simulink library "Lib_Piccolo"  (R2018b)
settings: Solver=VariableStepAuto  StartTime=0.0  StopTime=10.0  RelTol=1e-3
values from neighbouring files (symbols this model uses):
  AccelErrInt2Brakes = 0.15    [SimulationControlConfig16P.m]    (also in SimulationControlConfig16P_F0.m; SimulationControlConfig16P_F2.m; SimulationControlConfig16P_LEGACY.m; SimulationControlConfigTAILLESS.m = 0.2)
  AileronMax = 25    [SimulationControlConfig16P.m]    (also in SimulationControlConfig16P_F0.m; SimulationControlConfig16P_F2.m; SimulationControlConfig16P_LEGACY.m; SimulationControlConfigTAILLESS.m)
  AileronPower = 0.00268    [SimulationControlConfig16P.m]    (also in SimulationControlConfig16P_F0.m; SimulationControlConfig16P_F2.m; SimulationControlConfig16P_LEGACY.m; SimulationControlConfigTAILLESS.m = 0.002266)
  AileronSurfaceMax = 45    [SimulationControlConfig16P.m]    (also in SimulationControlConfig16P_F0.m; SimulationControlConfig16P_F2.m; SimulationControlConfig16P_LEGACY.m; SimulationControlConfigTAILLESS_CGAFT_F0.m = 25)
  AileronTrim = 0    [SimulationControlConfig16P.m]    (also in SimulationControlConfig16P_F0.m; SimulationControlConfig16P_F2.m; SimulationControlConfig16P_LEGACY.m; SimulationControlConfigTAILLESS.m)
  Alt = 1000 + TerrainHeight    [SimulationStateConfig.m]
  AltCruise_m = Alt * 0.3048    [SimulationControlConfig16P.m]    (also in SimulationControlConfig16P_F2.m; SimulationControlConfigTAILLESS.m = Alt/3.28084; SimulationControlConfigTAILLESS_CGAFT_F0.m = 640; SimulationControlConfigTAILLESS_CGFWD_F0.m = 640)
  AltitudeRate2PitchCmdIntegratorInit = 0.1    [SimulationControlPre.m]
  AltMax = 10000    [SimulationControlConfig16P.m]    (also in SimulationControlConfig16P_F0.m; SimulationControlConfig16P_F2.m; SimulationControlConfig16P_LEGACY.m; SimulationControlConfigTAILLESS.m)
  AltMaxAccel = 2.5    [SimulationControlConfig16P.m]    (also in SimulationControlConfig16P_F0.m = 2; SimulationControlConfig16P_F2.m = 2; SimulationControlConfig16P_LEGACY.m = 0.9; SimulationControlConfigTAILLESS.m = 2)
  AltMin = 0    [SimulationControlConfig16P.m]    (also in SimulationControlConfig16P_F0.m; SimulationControlConfig16P_F2.m; SimulationControlConfig16P_LEGACY.m; SimulationControlConfigTAILLESS.m)
  AltRateCmd2Pitch = 0.26    [SimulationControlConfig16P.m]    (also in SimulationControlConfig16P_F0.m = 0.35; SimulationControlConfig16P_F2.m = 0.35; SimulationControlConfig16P_LEGACY.m = 0.6; SimulationControlConfigTAILLESS.m = 0.9)
  AltRateError2Pitch = 0.34    [SimulationControlConfig16P.m]    (also in SimulationControlConfig16P_F0.m = 0.61; SimulationControlConfig16P_F2.m = 0.61; SimulationControlConfig16P_LEGACY.m = 0.4; SimulationControlConfigTAILLESS.m = 0.3)
  AltRateErrorInt2Pitch = 0.61    [SimulationControlConfig16P.m]    (also in SimulationControlConfig16P_F0.m = 0.28; SimulationControlConfig16P_F2.m = 0.28; SimulationControlConfig16P_LEGACY.m = 0.45; SimulationControlConfigTAILLESS.m = 0.15)
  AltRateLpfCutOff = 3    [SimulationControlConfig16P.m]    (also in SimulationControlConfig16P_F0.m; SimulationControlConfig16P_F2.m; SimulationControlConfig16P_LEGACY.m; SimulationControlConfigTAILLESS.m = 5)
  AutoNosegear2Rudder = 26    [SimulationControlConfig16P.m]    (also in SimulationControlConfig16P_F0.m; SimulationControlConfig16P_F2.m; SimulationControlConfig16P_LEGACY.m; SimulationControlConfigTAILLESS.m = 25.2)
  b = 5.54    [SimulationControlConfig16P.m]    (also in SimulationControlConfig16P_F0.m; SimulationControlConfig16P_F2.m; SimulationControlConfig16P_LEGACY.m; SimulationControlConfigTAILLESS.m = 2.37)
  Bank2AileronIntegratorInit = 0    [SimulationControlPre.m]
  BankMax_User = BankMax_User/180*pi    (= 0.610865238198)    [SimulationControlConfig16P.m]    (also in SimulationControlConfig16P_F0.m = 0.523598775598; SimulationControlConfig16P_F2.m = 0.523598775598; SimulationControlConfig16P_LEGACY.m = 0.523598775598; SimulationControlConfigTAILLESS.m = 0.558505360638)
  baseLegFlaps = 20    [SimulationControlConfig16P.m]    (also in SimulationControlConfig16P_F0.m; SimulationControlConfig16P_F2.m = 15; SimulationControlConfig16P_LEGACY.m = 0; SimulationControlConfigTAILLESS.m = 0)
  C = GeneticOpt.C    [SimulationCostFunction.m]
  c = Sw/b    (= 0.841696750903)    [SimulationControlConfig16P.m]    (also in SimulationControlConfig16P_F0.m; SimulationControlConfig16P_F2.m; SimulationControlConfig16P_LEGACY.m; SimulationControlConfigTAILLESS.m = 0.354008438819)
  cell2WheelFactorMG = 5.98    [SimulationSensorConfig16P_LEGACY.m]
  cell2WheelFactorNG = 1    [SimulationSensorConfig16P_LEGACY.m]
  cellSatMaxMG = 15000    [SimulationSensorConfig16P.m]    (also in SimulationSensorConfig16P_LEGACY.m; SimulationSensorConfigTAILLESS7P.m; SimulationSensorConfigUTAIL7P.m)
  cellSatMaxNG = 1000    [SimulationSensorConfig16P.m]    (also in SimulationSensorConfig16P_LEGACY.m; SimulationSensorConfigTAILLESS7P.m; SimulationSensorConfigUTAIL7P.m)
  cellSatMinMG = -15000    [SimulationSensorConfig16P.m]    (also in SimulationSensorConfig16P_LEGACY.m; SimulationSensorConfigTAILLESS7P.m; SimulationSensorConfigUTAIL7P.m)
  cellSatMinNG = -1000    [SimulationSensorConfig16P.m]    (also in SimulationSensorConfig16P_LEGACY.m; SimulationSensorConfigTAILLESS7P.m; SimulationSensorConfigUTAIL7P.m)
  CL_Limit = CL_Max    (= 0.54)    [SimulationControlConfig16P.m]    (also in SimulationControlConfig16P_F0.m; SimulationControlConfig16P_F2.m = 0.638; SimulationControlConfig16P_LEGACY.m; SimulationControlConfigTAILLESS.m = 0.525)
  CL_Max = 0.54    [SimulationControlConfig16P.m]    (also in SimulationControlConfig16P_F0.m; SimulationControlConfig16P_F2.m = 0.638; SimulationControlConfig16P_LEGACY.m; SimulationControlConfigTAILLESS.m = 0.525)
  CL_Max_Nom = 0.465    [SimulationControlConfig16P.m]    (also in SimulationControlConfig16P_F0.m; SimulationControlConfig16P_F2.m = 0.563; SimulationControlConfig16P_LEGACY.m; SimulationControlConfigTAILLESS.m = 0.39)
  CL_Min = 0    [SimulationControlConfig16P.m]    (also in SimulationControlConfig16P_F0.m; SimulationControlConfig16P_F2.m; SimulationControlConfig16P_LEGACY.m; SimulationControlConfigTAILLESS.m)
  ClimbMaxFraction = 0.35    [SimulationControlConfig16P.m]    (also in SimulationControlConfig16P_F0.m = 0.17; SimulationControlConfig16P_F2.m = 0.17; SimulationControlConfig16P_LEGACY.m = 0.24; SimulationControlConfigTAILLESS.m = 0.21)
  ClimboutMaxBank = 7.0    (= 7)    [SimulationControlConfig16P.m]    (also in SimulationControlConfig16P_F0.m; SimulationControlConfig16P_F2.m; SimulationControlConfig16P_LEGACY.m; SimulationControlConfigTAILLESS.m = 5)
  ClimboutTimer = 7.0    (= 7)    [SimulationControlConfig16P.m]    (also in SimulationControlConfig16P_F0.m; SimulationControlConfig16P_F2.m; SimulationControlConfig16P_LEGACY.m; SimulationControlConfigTAILLESS.m)
  dCl_per_dFlap = 0.005581818    [SimulationControlConfig16P.m]    (also in SimulationControlConfig16P_F0.m = 0; SimulationControlConfig16P_F2.m = 0.0065; SimulationControlConfig16P_LEGACY.m = 0; SimulationControlConfigTAILLESS.m = 0)
  DecelerationCmd = 3.1    [SimulationControlConfig16P.m]    (also in SimulationControlConfig16P_F0.m; SimulationControlConfig16P_F2.m; SimulationControlConfig16P_LEGACY.m; SimulationControlConfigTAILLESS.m = 0.1)
  DeRotateLogicEndTimer = abs((NoseDownLimit_Deg-1)/DeRotateRamp_Dps)    [SimulationControlConfig16P.m]    (also in SimulationControlConfig16P_F0.m; SimulationControlConfig16P_F2.m; SimulationControlConfig16P_LEGACY.m; SimulationControlConfigTAILLESS.m)
  DeRotateLogicHoldNoseUpTimer = 0.1    [SimulationControlConfig16P.m]    (also in SimulationControlConfig16P_F0.m; SimulationControlConfig16P_F2.m; SimulationControlConfig16P_LEGACY.m; SimulationControlConfigTAILLESS.m)
  DeRotateLogicTimerTimeout = 2    [SimulationControlConfig16P.m]    (also in SimulationControlConfig16P_F0.m; SimulationControlConfig16P_F2.m; SimulationControlConfig16P_LEGACY.m; SimulationControlConfigTAILLESS.m)
  DeRotateLowerCmdSaturation = 0    [SimulationControlConfig16P.m]    (also in SimulationControlConfig16P_F0.m; SimulationControlConfig16P_F2.m; SimulationControlConfig16P_LEGACY.m; SimulationControlConfigTAILLESS.m)
  DeRotateRamp_Dps = 3    [SimulationControlConfig16P.m]    (also in SimulationControlConfig16P_F0.m; SimulationControlConfig16P_F2.m; SimulationControlConfig16P_LEGACY.m; SimulationControlConfigTAILLESS.m = 8)
  DeRotateUpperCmdSaturation = 7    [SimulationControlConfig16P.m]    (also in SimulationControlConfig16P_F0.m; SimulationControlConfig16P_F2.m; SimulationControlConfig16P_LEGACY.m; SimulationControlConfigTAILLESS.m)
  DescentMaxFraction = 0.22    [SimulationControlConfig16P.m]    (also in SimulationControlConfig16P_F0.m = 0.2; SimulationControlConfig16P_F2.m = 0.2; SimulationControlConfig16P_LEGACY.m = 0.2; SimulationControlConfigTAILLESS.m = 0.17)
  DesktopSimTerrainOffset_m = 0.406    [SimulationAircraftConfig.m]
  downwindFlaps = 0    [SimulationControlConfig16P.m]    (also in SimulationControlConfig16P_F0.m; SimulationControlConfig16P_F2.m = 15; SimulationControlConfig16P_LEGACY.m; SimulationControlConfigTAILLESS.m)
  downwindSplitAil = 0    [SimulationControlConfig16P_F2.m]
  DP_init = 0.5*1.225*V_init^2    [SimulationControlConfig16P.m]    (also in SimulationControlConfig16P_F0.m; SimulationControlConfig16P_F2.m; SimulationControlConfig16P_LEGACY.m; SimulationControlConfigTAILLESS.m)
  dscNoiseMG = 1    [SimulationSensorConfig16P_LEGACY.m]
  dscNoiseNG = 0.25    [SimulationSensorConfig16P_LEGACY.m]
  DSCnumBits = 24    [SimulationSensorConfig16P.m]    (also in SimulationSensorConfig16P_LEGACY.m; SimulationSensorConfigTAILLESS7P.m; SimulationSensorConfigUTAIL7P.m)
  DSCRangeMaxMG = 15000    [SimulationSensorConfig16P.m]    (also in SimulationSensorConfig16P_LEGACY.m; SimulationSensorConfigTAILLESS7P.m; SimulationSensorConfigUTAIL7P.m)
  DSCRangeMaxNG = 1000    [SimulationSensorConfig16P.m]    (also in SimulationSensorConfig16P_LEGACY.m; SimulationSensorConfigTAILLESS7P.m; SimulationSensorConfigUTAIL7P.m)
  DSCRangeMinMG = -15000    [SimulationSensorConfig16P.m]    (also in SimulationSensorConfig16P_LEGACY.m; SimulationSensorConfigTAILLESS7P.m; SimulationSensorConfigUTAIL7P.m)
  DSCRangeMinNG = -1000    [SimulationSensorConfig16P.m]    (also in SimulationSensorConfig16P_LEGACY.m; SimulationSensorConfigTAILLESS7P.m; SimulationSensorConfigUTAIL7P.m)
  dt = DLLSim.dt    [SimulationTimeStep.m]    (also in SimulationTrim.m = 0.02)
  EarlyTouchdownThreshold = 3.0    (= 3)    [SimulationControlConfig16P.m]    (also in SimulationControlConfig16P_F0.m; SimulationControlConfig16P_F2.m; SimulationControlConfig16P_LEGACY.m; SimulationControlConfigTAILLESS.m)
  ElevatorDeflectionRate = 15    [SimulationControlConfig16P.m]    (also in SimulationControlConfig16P_F0.m; SimulationControlConfig16P_F2.m; SimulationControlConfig16P_LEGACY.m = 12; SimulationControlConfigTAILLESS.m = 5)
  ElevatorMax = 25    [SimulationControlConfig16P.m]    (also in SimulationControlConfig16P_F0.m; SimulationControlConfig16P_F2.m; SimulationControlConfig16P_LEGACY.m; SimulationControlConfigTAILLESS.m)
  ElevatorPower = -0.002209    [SimulationControlConfig16P.m]    (also in SimulationControlConfig16P_F0.m; SimulationControlConfig16P_F2.m; SimulationControlConfig16P_LEGACY.m; SimulationControlConfigTAILLESS.m = -0.002668)
  ElevatorTrim = -3.5    [SimulationControlConfig16P.m]    (also in SimulationControlConfig16P_F0.m; SimulationControlConfig16P_F2.m; SimulationControlConfig16P_LEGACY.m; SimulationControlConfigTAILLESS.m = -3)
  elevonBias = 0    [SimulationControlConfig16P.m]    (also in SimulationControlConfig16P_F0.m; SimulationControlConfig16P_F2.m; SimulationControlConfig16P_LEGACY.m; SimulationControlConfigTAILLESS.m)
  Enable_TAS_Protection = 0    [SimulationControlConfig16P.m]    (also in SimulationControlConfig16P_F0.m; SimulationControlConfig16P_F2.m; SimulationControlConfig16P_LEGACY.m; SimulationControlConfigTAILLESS.m)
  EnableCrossTrackAbort = 1    [SimulationControlConfig16P.m]    (also in SimulationControlConfigTAILLESS.m; SimulationControlConfigTAILLESS_CGAFT_F0.m; SimulationControlConfigTAILLESS_CGFWD_F0.m; SimulationControlConfigTAILLESS_CGFWD_F2.m)
  EnergyBandwidth = 0.04    [SimulationControlConfig16P.m]    (also in SimulationControlConfig16P_F0.m = 0.03; SimulationControlConfig16P_F2.m = 0.03; SimulationControlConfig16P_LEGACY.m = 0.02; SimulationControlConfigTAILLESS.m = 0.06)
  EngineLhFuelCut = 0    [SimulationAircraftConfig.m]
  EngineRhFuelCut = 0    [SimulationAircraftConfig.m]
  FastThrottleRate = 0.075    [SimulationControlConfig16P.m]    (also in SimulationControlConfig16P_F0.m = 0.05; SimulationControlConfig16P_F2.m = 0.05; SimulationControlConfig16P_LEGACY.m = 0.05; SimulationControlConfigTAILLESS.m = 0.1)
  FilterWarmUpTime = 2    [SimulationSensorConfig16P.m]    (also in SimulationSensorConfig16P_LEGACY.m; SimulationSensorConfigTAILLESS7P.m; SimulationSensorConfigUTAIL7P.m)
  finalApproachFlaps = 20    [SimulationControlConfig16P.m]    (also in SimulationControlConfig16P_F0.m; SimulationControlConfig16P_F2.m = 15; SimulationControlConfig16P_LEGACY.m = 0; SimulationControlConfigTAILLESS.m = 0)
  finalApproachSplitAil = 20    [SimulationControlConfig16P_F2.m]
  FinalDescentSlope_Deg = testPlans(testIndx).descentSlope    [SimulationControlConfig16P.m]    (also in SimulationControlConfig16P_F0.m; SimulationControlConfig16P_F2.m; SimulationControlConfig16P_LEGACY.m; SimulationControlConfigTAILLESS.m)
  flapMax = 0    [SimulationControlConfig16P.m]    (also in SimulationControlConfig16P_F0.m = 35; SimulationControlConfig16P_F2.m = 33; SimulationControlConfig16P_LEGACY.m; SimulationControlConfigTAILLESS.m)
  flapRate = 7.5    [SimulationControlConfig16P.m]    (also in SimulationControlConfig16P_F0.m; SimulationControlConfig16P_F2.m; SimulationControlConfig16P_LEGACY.m; SimulationControlConfigTAILLESS.m = 6.6)
  FlareHeight = 5    [SimulationControlConfig16P.m]    (also in SimulationControlConfig16P_F0.m; SimulationControlConfig16P_F2.m; SimulationControlConfig16P_LEGACY.m = 4.8; SimulationControlConfigTAILLESS.m = 2.75)
  FlareVerticalRate_mps = -0.4    [SimulationControlConfig16P.m]    (also in SimulationControlConfig16P_F0.m; SimulationControlConfig16P_F2.m; SimulationControlConfig16P_LEGACY.m = -0.5; SimulationControlConfigTAILLESS.m = -0.15)
  Fp_Aileron = 0.55*2*pi*RollRateLpfCutoff*dt    [SimulationControlConfig16P.m]    (also in SimulationControlConfig16P_F0.m; SimulationControlConfig16P_F2.m; SimulationControlConfig16P_LEGACY.m; SimulationControlConfigTAILLESS.m)
  Fp_Alt = 2*pi*0.55*AltBandwidth    (= 0.622035345411)    [SimulationControlConfig16P.m]    (also in SimulationControlConfig16P_F0.m; SimulationControlConfig16P_F2.m; SimulationControlConfig16P_LEGACY.m = 0.099; SimulationControlConfigTAILLESS.m = 0.207345115137)
  Fp_AltRate = 0.55*2*pi*AltRateLpfCutOff*dt    [SimulationControlConfig16P.m]    (also in SimulationControlConfig16P_F0.m; SimulationControlConfig16P_F2.m; SimulationControlConfig16P_LEGACY.m; SimulationControlConfigTAILLESS.m)
  Fp_Elevator = 0.55*2*pi*PitchRateLpfCutoff*dt    [SimulationControlConfig16P.m]    (also in SimulationControlConfig16P_F0.m; SimulationControlConfig16P_F2.m; SimulationControlConfig16P_LEGACY.m; SimulationControlConfigTAILLESS.m)
  Fp_Energy = 0.55*2*pi*EnergyBandwidth    (= 0.138230076758)    [SimulationControlConfig16P.m]    (also in SimulationControlConfig16P_F0.m = 0.103672557568; SimulationControlConfig16P_F2.m = 0.103672557568; SimulationControlConfig16P_LEGACY.m = 0.069115038379; SimulationControlConfigTAILLESS.m = 0.207345115137)
  Fp_Energy2 = 0.55*2*pi*EnergyBandwidth*dt    [SimulationControlConfig16P.m]    (also in SimulationControlConfig16P_F0.m; SimulationControlConfig16P_F2.m; SimulationControlConfig16P_LEGACY.m; SimulationControlConfigTAILLESS.m)
  Fp_Pitch = 0.55*2*pi*PitchBandwidth    (= 2.45358386245)    [SimulationControlConfig16P.m]    (also in SimulationControlConfig16P_F0.m; SimulationControlConfig16P_F2.m = 1.72787595947; SimulationControlConfig16P_LEGACY.m = 3.11017672705; SimulationControlConfigTAILLESS.m = 1.55508836353)
  Fp_Pitch_2 = 0.55*2*pi*PitchBandwidth*dt    [SimulationControlConfig16P.m]    (also in SimulationControlConfig16P_F0.m; SimulationControlConfig16P_F2.m; SimulationControlConfig16P_LEGACY.m; SimulationControlConfigTAILLESS.m)
  Fp_Roll = RollBandwidth^2    (= 1.69)    [SimulationControlConfig16P.m]    (also in SimulationControlConfig16P_F0.m = 1.44; SimulationControlConfig16P_F2.m = 1.44; SimulationControlConfig16P_LEGACY.m = 1.44; SimulationControlConfigTAILLESS.m = 1.21)
  Fp_Rudder = 0.55*2*pi*YawRateLpfCutoff*dt    [SimulationControlConfig16P.m]    (also in SimulationControlConfig16P_F0.m; SimulationControlConfig16P_F2.m; SimulationControlConfig16P_LEGACY.m; SimulationControlConfigTAILLESS.m)
  Fp_TAS = 0.55*2*pi*TASBandwidth    (= 0.103672557568)    [SimulationControlConfig16P.m]    (also in SimulationControlConfig16P_F0.m; SimulationControlConfig16P_F2.m; SimulationControlConfig16P_LEGACY.m; SimulationControlConfigTAILLESS.m = 0.172787595947)
  Fp_TAS_Filter = 2*pi*TasLpfCutoff*dt    [SimulationControlConfig16P.m]    (also in SimulationControlConfig16P_F0.m; SimulationControlConfig16P_F2.m; SimulationControlConfig16P_LEGACY.m; SimulationControlConfigTAILLESS.m)
  Fp_Turn = 0.55*2*pi*TurnErrLPFcutoff    (= 0.172787595947)    [SimulationControlConfig16P.m]    (also in SimulationControlConfig16P_F0.m = 0.0345575191895; SimulationControlConfig16P_F2.m = 0.0345575191895; SimulationControlConfig16P_LEGACY.m = 0.0345575191895; SimulationControlConfigTAILLESS.m)
  Fp_TurnDerr = 0.55*2*pi*TurnDerivativeLPFcutoff    (= 0.172787595947)    [SimulationControlConfig16P.m]    (also in SimulationControlConfig16P_F0.m = 0.0345575191895; SimulationControlConfig16P_F2.m = 0.0345575191895; SimulationControlConfig16P_LEGACY.m = 0.0345575191895; SimulationControlConfigTAILLESS.m)
  FTV = 3    [SimulationAircraftConfig.m]
  ftvStaticPositionError = 1/1.18    (= 0.847457627119)    [SimulationSensorConfig16P.m]    (also in SimulationSensorConfig16P_LEGACY.m; SimulationSensorConfigTAILLESS7P.m = 1; SimulationSensorConfigUTAIL7P.m = 1)
  g = 9.81    [SimulationStateConfig.m]
  goAroundSplitAil = 0    [SimulationControlConfig16P_F2.m]
  GustSpd_Kts = testPlans(testIndx).gustSpd    [SimulationStateConfig.m]
  GustTriggerVal = testPlans(testIndx).gustTriggerVal    [SimulationStateConfig.m]
  HeadingErr2TurnRate = 0.5    [SimulationControlConfig16P.m]    (also in SimulationControlConfig16P_F0.m; SimulationControlConfig16P_F2.m; SimulationControlConfig16P_LEGACY.m; SimulationControlConfigTAILLESS.m)
  HeadingErrDer2TurnRate = 0.3    [SimulationControlConfig16P.m]    (also in SimulationControlConfig16P_F0.m; SimulationControlConfig16P_F2.m; SimulationControlConfig16P_LEGACY.m; SimulationControlConfigTAILLESS.m)
  IASbounce = IASstall*0.8    [SimulationControlPre.m]
  IAScruiseCMD = sqrt(2*m*9.81/(1.225*Sw*CL_cruise))    [SimulationControlConfig16P.m]    (also in SimulationControlConfig16P_F0.m; SimulationControlConfig16P_F2.m; SimulationControlConfig16P_LEGACY.m; SimulationControlConfigTAILLESS.m)
  IASfinalCMD = 1.12 * IASmin    [SimulationControlConfig16P.m]    (also in SimulationControlConfig16P_F0.m = 1.14 * IASmin; SimulationControlConfig16P_F2.m = 1.10 * IASmin; SimulationControlConfig16P_LEGACY.m = 1.10 * IASmin; SimulationControlConfigTAILLESS.m = 1.14 * IASmin)
  IASflareCMD = IASstall    [SimulationControlConfig16P.m]    (also in SimulationControlConfig16P_F0.m; SimulationControlConfig16P_F2.m; SimulationControlConfig16P_LEGACY.m; SimulationControlConfigTAILLESS.m)
  IASmax = 64    [SimulationControlConfig16P.m]    (also in SimulationControlConfig16P_F0.m = 46; SimulationControlConfig16P_F2.m = 52; SimulationControlConfig16P_LEGACY.m = 46; SimulationControlConfigTAILLESS.m = 38.9)
  IASmin = sqrt(2*m*9.81/(1.225*Sw*0.9*CL_Max_Nom))    [SimulationControlConfig16P.m]    (also in SimulationControlConfig16P_F0.m; SimulationControlConfig16P_F2.m; SimulationControlConfig16P_LEGACY.m; SimulationControlConfigTAILLESS.m)
  IASshortCMD = IASstall    [SimulationControlConfig16P.m]    (also in SimulationControlConfig16P_F0.m; SimulationControlConfig16P_F2.m; SimulationControlConfig16P_LEGACY.m; SimulationControlConfigTAILLESS.m)
  IASstall = sqrt(2*m*9.81/(1.225*Sw*CL_Max))    [SimulationControlConfig16P.m]    (also in SimulationControlConfig16P_F0.m; SimulationControlConfig16P_F2.m; SimulationControlConfig16P_LEGACY.m; SimulationControlConfigTAILLESS.m)
  inFlight = 1    [SimulationControlConfig16P.m]    (also in SimulationControlConfigTAILLESS.m; SimulationControlConfigTAILLESS_CGAFT_F0.m; SimulationControlConfigTAILLESS_CGFWD_F0.m; SimulationControlConfigTAILLESS_CGFWD_F2.m)
  JetCatOffset = 5    [SimulationControlConfig16P.m]    (also in SimulationControlConfig16P_F0.m; SimulationControlConfig16P_F2.m; SimulationControlConfig16P_LEGACY.m)
  LaunchRollingElevator = -1.5    [SimulationControlConfig16P.m]    (also in SimulationControlConfig16P_F0.m; SimulationControlConfig16P_F2.m = 1.25; SimulationControlConfig16P_LEGACY.m; SimulationControlConfigTAILLESS.m = 1)
  ldg_NosegearMax = 10    [SimulationControlConfig16P.m]    (also in SimulationControlConfig16P_F0.m; SimulationControlConfig16P_F2.m; SimulationControlConfig16P_LEGACY.m; SimulationControlConfigTAILLESS.m)
  ldg_TrackVyErrInt2Nosegear = 0.1250    (= 0.125)    [SimulationControlConfig16P.m]    (also in SimulationControlConfig16P_F0.m; SimulationControlConfig16P_F2.m; SimulationControlConfig16P_LEGACY.m; SimulationControlConfigTAILLESS.m = 0.00714285714286)
  ldg_TrackVyErrPro2Nosegear = 0.35    [SimulationControlConfig16P.m]    (also in SimulationControlConfig16P_F0.m; SimulationControlConfig16P_F2.m; SimulationControlConfig16P_LEGACY.m; SimulationControlConfigTAILLESS.m = 0.0546666666667)
  ldg_TrackY2Vy = 0.07    [SimulationControlConfig16P.m]    (also in SimulationControlConfig16P_F0.m; SimulationControlConfig16P_F2.m; SimulationControlConfig16P_LEGACY.m; SimulationControlConfigTAILLESS.m = 0.17)
  ldg_Vy2NosegearScalingPower = 1.075    [SimulationControlConfig16P.m]    (also in SimulationControlConfig16P_F0.m; SimulationControlConfig16P_F2.m; SimulationControlConfig16P_LEGACY.m; SimulationControlConfigTAILLESS.m = 0.6)
  ldg_Y2VyScalingPower = 0.175    [SimulationControlConfig16P.m]    (also in SimulationControlConfig16P_F0.m; SimulationControlConfig16P_F2.m; SimulationControlConfig16P_LEGACY.m; SimulationControlConfigTAILLESS.m = 0)
  ldg_YawRate2Nosegear = 0.175    [SimulationControlConfig16P.m]    (also in SimulationControlConfig16P_F0.m; SimulationControlConfig16P_F2.m; SimulationControlConfig16P_LEGACY.m; SimulationControlConfigTAILLESS.m = 0.065)
  LiftSlope = 0.064285    [SimulationControlConfig16P.m]    (also in SimulationControlConfig16P_F0.m; SimulationControlConfig16P_F2.m; SimulationControlConfig16P_LEGACY.m; SimulationControlConfigTAILLESS.m = 0.058631)
  LPFaileronInit = 0    [SimulationControlPre.m]
  LPFclestInit = 0    [SimulationControlPre.m]
  LPFenergyFFInit = 0    [SimulationControlPre.m]
  ... (+122 more)
undefined symbols (not defined in the file or in its folder): abortFlag, alphaHPF, apmDelay, BRWNOUT, CRAWOR, CRAWUR, DiscIntNeverNeededParam, DLLSim, DLLSimStep, ECOMOR, ECOMUR, Fp_Tas, GustTrigger_HeightAgl_m, IPSTAT, LCINTEG, Ldg_Persist_Time, LOWER_FLAGS, MSG_ENABLE, NoiseStd, OLDVAL, OVERRIDE_ENABLE, OVERRIDE_VALUE, REBOOT, reversionEnable, revIASMax, revIASMin, revPitchMax, revPitchMin, revPitchRateMax, revRollMax, revRollRateMax, SAMPLE, SCALON, SensorModel, sigbuilder_block, Sim_Vx, Sim_Vy, Sim_Vz, Sim_Xpos, Sim_Ypos, Sim_Zpos, SYSOR, SYSUR, TARE, TEMPOR, TEMPUR, testIndx, testPlan, testPlans, Trim_piccoloInCmd, Trim_REFSI_FD_IN_nmodeCgShifterCmd_Flag, Trim_REFSI_FD_IN_nmodeCgShifterCmd_Ft, Trim_REFSI_FD_IN_nmodeCgShifterCmdType, Trim_REFSI_FD_IN_nmodeCgShifterNRCActive, Trim_REFSI_FD_IN_nmodeFlapLhIBCmd_Deg, Trim_REFSI_FD_IN_nmodeFlapLhOBCmd_Deg, Trim_REFSI_FD_IN_nmodeFlapRhIBCmd_Deg, Trim_REFSI_FD_IN_nmodeFlapRhOBCmd_Deg, Trim_REFSI_FD_IN_nmodeSlatLhCmd_Deg ... (+11)
libraries: simulink x1237, $bdroot x179, aerolibconvert2 x63, dspswit3 x25, aerolibatmos2 x5, simulink_extras x4, dsparch4 x2, Lib_Piccolo_Alt x2, eeGeneralControl x1, dspindex x1
(part 14 of 74)

== system Lib_Piccolo/Piccolo State Machine/Flight State Machine ==
  <apMode> : Inport
  IAS : Inport  Port=2
  GroundSpeed : Inport  Port=3
  AND : Logic  IconShape=distinctive  AllPortsSameDT=off  OutDataTypeStr=boolean
  AND1 : Logic  IconShape=distinctive  AllPortsSameDT=off  OutDataTypeStr=boolean
  Abort Logic : Subsystem
  Compare To Constant : simulink/Logic and Bit Operations/Compare To Constant  relop===  const=0  OutDataTypeStr=boolean
  Compare To Constant1 : simulink/Logic and Bit Operations/Compare To Constant  relop===  const=3.0  OutDataTypeStr=boolean
  Compare To Constant2 : simulink/Logic and Bit Operations/Compare To Constant  relop=>=  const=ClimboutTimer  OutDataTypeStr=boolean
  Compare To Constant3 : simulink/Logic and Bit Operations/Compare To Constant  relop=>=  const=0.75*IASmin  OutDataTypeStr=boolean
  Compare To Constant4 : simulink/Logic and Bit Operations/Compare To Constant  relop=>=  const=RotationSpeed  OutDataTypeStr=boolean
  Constant : Constant  Value=2
  Constant{1,3,5..6} (4 alike) : Constant
  Constant2 : Constant  Value=3
  Constant4 : Constant  Value=4
  Constant9 : Constant  Value=11
  Latch : Subsystem
  Latch1 : Subsystem
  Latch2 : Subsystem
  Switch{,1..3} (4 alike) : Switch  Criteria=u2 > Threshold
  Switch4 : Switch  Criteria=u2 > Threshold  Threshold=0.5
  Timer : Subsystem  mask{period=3}
      mask prompts: period "Period [s]"
  Unit Delay : UnitDelay  SampleTime=-1
  Unit Delay1 : UnitDelay  SampleTime=-1
  Sim.apMode : Outport
  tag scope: RotationFlag=global, TakeoffAbortFlag=global
  wires:
  GroundSpeed/1 -> Abort Logic/2(GroundSpeed)
  <apMode>/1 -> Switch3/3
  Constant/1 -> Switch/1
  Constant1/1 -> Latch/2(Enable/!Rst)
  [RotationFlag] -> AND1/1
  Latch/1(Q_Latched) -> Switch/2
  [TouchdownDetectedFlag] -> Compare To Constant/1
  Latch2/1(Q_Latched) -> Switch1/2
  Switch/1 -> Switch1/3
  Constant2/1 -> Switch1/1
  Compare To Constant1/1 -> Timer/1(Run/!Reset)
  Switch1/1 -> Compare To Constant1/1, Switch2/3
  Timer/1(timeOut_s) -> Compare To Constant2/1
  Compare To Constant2/1 -> Latch1/1(D)
  Constant3/1 -> Latch1/2(Enable/!Rst)
  Latch1/1(Q_Latched) -> Switch2/2
  Switch2/1 -> Switch4/3
  Constant4/1 -> Switch2/1
  Compare To Constant/1 -> AND/2
  Compare To Constant3/1 -> AND/1
  AND/1 -> Latch2/1(D)
  Constant5/1 -> Latch2/2(Enable/!Rst)
  Switch3/1 -> Switch/3
  Constant6/1 -> Switch3/1
  [startTaxi] -> AND1/2, Switch3/2
  AND1/1 -> Latch/1(D)
  IAS/1 -> Unit Delay/1, Abort Logic/1(IAS), Compare To Constant3/1
  Compare To Constant4/1 -> [RotationFlag]  "RotationFlag"
  Unit Delay/1 -> Compare To Constant4/1
  Switch4/1 -> Unit Delay1/1
  [TakeoffAbortFlag] -> Switch4/2
  Constant9/1 -> Switch4/1
  Abort Logic/1(Flag_TakeoffAbort) -> [TakeoffAbortFlag]
  Unit Delay1/1 -> Sim.apMode/1

== system Lib_Piccolo/Piccolo State Machine/Landing State Machine ==
  note: Moved to Vertical Track Following Guidance in Next Block
  <apMode> : Inport
  Compare To Constant1 : simulink/Logic and Bit Operations/Compare To Constant  relop=>  const=0  OutDataTypeStr=boolean
  Compare To Constant3 : simulink/Logic and Bit Operations/Compare To Constant  relop=>  const=0  OutDataTypeStr=boolean
  Constant : Constant  Value=9
  Constant1 : Constant  Value=10
  Constant2 : Constant  Value=11
  Constant3 : Constant  Value=8
  Flare Detection : Subsystem
  FlareLatch : Subsystem
  NOT1 : Logic  Operator=NOT  IconShape=distinctive  AllPortsSameDT=off  OutDataTypeStr=boolean
  NOT2 : Logic  Operator=NOT  IconShape=distinctive  AllPortsSameDT=off  OutDataTypeStr=boolean
  ShortFinal Detection : Subsystem  Commented=on
  Switch{,1..3} (4 alike) : Switch  Criteria=u2 > Threshold
  Sim.apMode : Outport
  wires:
  Compare To Constant3/1 -> NOT2/1
  [FlareFlag] -> FlareLatch/2(FlareFlag)
  Constant3/1 -> Switch3/3
  Switch1/1 -> Switch2/1
  Switch2/1 -> Sim.apMode/1  "Sim.apMode"
  [ShortFinalFlag] -> Compare To Constant1/1
  <apMode>/1 -> Switch3/1
  Constant/1 -> Switch/3
  NOT2/1 -> Switch2/2
  [FinalFlag] -> NOT1/1
  Constant1/1 -> Switch1/3
  Switch/1 -> Switch1/1
  Switch3/1 -> Switch/1
  [Pic_AP_Mode] -> FlareLatch/1(apMode)
  [TouchdownDetectedFlag] -> Compare To Constant3/1
  FlareLatch/1(FlareLatch) -> Switch1/2
  Constant2/1 -> Switch2/3
  NOT1/1 -> Switch3/2
  Compare To Constant1/1 -> Switch/2

== system Lib_Piccolo/Piccolo State Machine FLIGHT LEGACY/Flare Detection ==
  Compare To Constant : simulink/Logic and Bit Operations/Compare To Constant  relop=>  const=0  OutDataTypeStr=boolean
  Delay : Delay  DelayLength=0.04/dt  InitialCondition=Alt*0.3048
  "FlareHeight_m " : Constant  Value=FlareHeight
  Sum : Sum  Inputs=|++
  Sum1 : Sum  Inputs=|+-
  Sum2 : Sum  Inputs=|++
  Sum4 : Sum  Inputs=|+-
  Sum5 : Sum  Inputs=|+-
  Terminator10 : Terminator
  "TerrainHeight " : Constant  Value=TerrainHeight
  VehicleRestingHeight : Constant  Value=DesktopSimTerrainOffset_m
  ft to m : Gain  Gain=0.3048
  tag scope: AltAGL_m=global, FlareFlag=global
  wires:
  Sum2/1 -> Sum1/2
  Sum1/1 -> Compare To Constant/1, [FlareFlag]
  VehicleRestingHeight/1 -> Sum2/2, Sum5/2
  ft to m/1 -> Sum4/2, Sum/1
  "TerrainHeight "/1 -> ft to m/1
  Sum5/1 -> [AltAGL_m]  "AltAGL_m"
  Sum4/1 -> Sum5/1
  Compare To Constant/1 -> Terminator10/1  "Sim.FlareFlag"
  "FlareHeight_m "/1 -> Sum/2
  [Alt_m] -> Delay/1, Sum4/1
  Delay/1 -> Sum1/1
  Sum/1 -> Sum2/1

== system Lib_Piccolo/Piccolo State Machine FLIGHT LEGACY/ShortFinal Detection ==
  Compare To Constant4 : simulink/Logic and Bit Operations/Compare To Constant  relop=>  const=0  OutDataTypeStr=boolean
  ShortFinalHeight : Constant  Value=ShortFinalHeight
  Sum3 : Sum  Inputs=|+-
  tag scope: ShortFinalFlag=global
  wires:
  Compare To Constant4/1 -> [ShortFinalFlag]  "Sim.ShortFinalFlag"
  ShortFinalHeight/1 -> Sum3/2
  [Alt_m] -> Sum3/1
  Sum3/1 -> Compare To Constant4/1

== system Lib_Piccolo/Piccolo State Machine LDG/Flare Detection ==
  Compare To Constant : simulink/Logic and Bit Operations/Compare To Constant  relop=>  const=0  OutDataTypeStr=boolean
  Delay : Delay  DelayLength=0.04/dt  InitialCondition=Alt*0.3048
  "FlareHeight_m " : Constant  Value=FlareHeight
  Sum : Sum  Inputs=|++
  Sum1 : Sum  Inputs=|+-
  Sum2 : Sum  Inputs=|++
  Sum4 : Sum  Inputs=|+-
  Sum5 : Sum  Inputs=|+-
  Terminator10 : Terminator
  "TerrainHeight " : Constant  Value=TerrainHeight
  VehicleRestingHeight : Constant  Value=DesktopSimTerrainOffset_m
  ft to m : Gain  Gain=0.3048
  tag scope: AltAGL_m=global, FlareFlag=global
  wires:
  Sum2/1 -> Sum1/2
  Sum1/1 -> Compare To Constant/1, [FlareFlag]
  VehicleRestingHeight/1 -> Sum2/2, Sum5/2
  ft to m/1 -> Sum4/2, Sum/1
  "TerrainHeight "/1 -> ft to m/1
  Sum5/1 -> [AltAGL_m]  "AltAGL_m"
  Sum4/1 -> Sum5/1
  Compare To Constant/1 -> Terminator10/1  "Sim.FlareFlag"
  "FlareHeight_m "/1 -> Sum/2
  [Alt_m] -> Delay/1, Sum4/1
  Delay/1 -> Sum1/1
  Sum/1 -> Sum2/1

== system Lib_Piccolo/Piccolo State Machine LDG/FlareLatch ==
  apMode : Inport
  FlareFlag : Inport  Port=2
  Compare To Constant1 : simulink/Logic and Bit Operations/Compare To Constant  relop=>=  const=6  OutDataTypeStr=boolean
  Compare To Constant2 : simulink/Logic and Bit Operations/Compare To Constant  relop=<  const=0  OutDataTypeStr=boolean
  Latch : Subsystem
  NOT3 : Logic  Operator=NOT  IconShape=distinctive  AllPortsSameDT=off  OutDataTypeStr=boolean
  OR : Logic  Operator=OR  IconShape=distinctive  AllPortsSameDT=off  OutDataTypeStr=boolean
  Unit Delay : UnitDelay  SampleTime=-1
  FlareLatch : Outport
  wires:
  Compare To Constant2/1 -> OR/1, Latch/1(D)
  OR/1 -> NOT3/1
  FlareFlag/1 -> Compare To Constant2/1
  Latch/1(Q_Latched) -> OR/2
  NOT3/1 -> FlareLatch/1
  apMode/1 -> Unit Delay/1
  Compare To Constant1/1 -> Latch/2(Enable/!Rst)
  Unit Delay/1 -> Compare To Constant1/1

== system Lib_Piccolo/Piccolo State Machine LDG/ShortFinal Detection ==
  Compare To Constant4 : simulink/Logic and Bit Operations/Compare To Constant  relop=>  const=0  OutDataTypeStr=boolean
  ShortFinalHeight : Constant  Value=ShortFinalHeight
  Sum3 : Sum  Inputs=|+-
  tag scope: ShortFinalFlag=global
  wires:
  Compare To Constant4/1 -> [ShortFinalFlag]  "Sim.ShortFinalFlag"
  ShortFinalHeight/1 -> Sum3/2
  [Alt_m] -> Sum3/1
  Sum3/1 -> Compare To Constant4/1

== system Lib_Piccolo/Pitch to Elevator/1st Order Reference Model ==
  PitchCmd_Body : Inport
  "Pitch_Body " : Inport  Port=2
  "Scalar " : Inport  Port=3
  "PitchRateCmd_Body " : Inport  Port=4
  "PitchRateLimit_Max " : Inport  Port=5
  " PitchRateLimit_Min " : Inport  Port=6
  apMode : Inport  Port=7
  PitchRate_Body : Inport  Port=8
  Constant : Constant  Value=PitchMaxAccel
  Constant1 : Constant  Value=0
  Constant2 : Constant  Value=100
  Fp_pitch : Gain  Gain=Fp_Pitch
  Gain1 : Gain  Gain=-1
  Gain2 : Gain  Gain=180/pi
  Gain3 : Gain  Gain=180/pi
  Gain4 : Gain  Gain=180/pi
  Manual Switch : ManualSwitch
  Multiply : Product
  NOT : Logic  Operator=NOT  IconShape=distinctive  AllPortsSameDT=off  OutDataTypeStr=boolean
  OR : Logic  Operator=OR  IconShape=distinctive  AllPortsSameDT=off  OutDataTypeStr=boolean
  OR1 : Logic  Operator=OR  IconShape=distinctive  AllPortsSameDT=off  OutDataTypeStr=boolean
  PitchRate Max Accel Limit : Subsystem
  PitchRateCMD Limit : Subsystem
  Sum : Sum  Inputs=|+-
  Sum1 : Sum  Inputs=|++
  Switch : Switch  Criteria=u2 > Threshold  Threshold=0.5
  Switch1 : Switch  Criteria=u2 > Threshold  Threshold=0.5
  Terminator1 : Terminator
  Terminator2 : Terminator
  Terminator3 : Terminator
  resetCondition : Subsystem
  resetCondition1 : $bdroot/Pitch to Elevator/1st Order Reference Model/resetCondition  SystemSampleTime=-1
  PitchRateCmd_Body : Outport
  tag scope: pitchRateLimitFlag=global
  wires:
  resetCondition1/1 -> NOT/1
  resetCondition/1(Reset) -> Switch/2
  apMode/1 -> resetCondition1/1, resetCondition/1(apMode)
  PitchRate Max Accel Limit/1(Y) -> PitchRateCmd_Body/1
  Switch/1 -> PitchRate Max Accel Limit/2(u)
  OR/1 -> [pitchRateLimitFlag]  "Sim.pitchRateLimitFlag"
  PitchRateCMD Limit/2(lowerFlag) -> OR/2
  PitchRateCMD Limit/1(upperFlag) -> OR/1
  PitchRate_Body/1 -> Switch/1
  PitchRateCMD Limit/3(y) -> Switch/3
  Gain3/1 -> Terminator3/1  "Sim.pitchRateLimit_Max"
  Gain4/1 -> Terminator2/1  "Sim.pitchRateLimit_Min"
  Gain2/1 -> Terminator1/1  "Sim.pitchRateCmd_noLimits"
  Sum1/1 -> Gain2/1, PitchRateCMD Limit/2(u)
  "PitchRateCmd_Body "/1 -> Manual Switch/1
  Constant1/1 -> Manual Switch/2
  Manual Switch/1 -> Sum1/2
  " PitchRateLimit_Min "/1 -> Gain4/1, PitchRateCMD Limit/3(lo)
  "PitchRateLimit_Max "/1 -> Gain3/1, PitchRateCMD Limit/1(up)
  Gain1/1 -> PitchRate Max Accel Limit/3(lo)
  Constant/1 -> Multiply/2
  Switch1/1 -> Gain1/1, PitchRate Max Accel Limit/1(up)
  "Scalar "/1 -> Multiply/1
  Fp_pitch/1 -> Sum1/1
  Sum/1 -> Fp_pitch/1
  "Pitch_Body "/1 -> Sum/2
  PitchCmd_Body/1 -> Sum/1
  Multiply/1 -> Switch1/1  "Sim.pitchMaxAccel"
  NOT/1 -> Switch1/2
  Constant2/1 -> Switch1/3
  PitchRate Max Accel Limit/2(upperFlag) -> OR1/1
  PitchRate Max Accel Limit/3(lowerFlag) -> OR1/2
  OR1/1 -> [pitchAccelLimitFlag]  "Sim.pitchAccelLimitFlag"

== system Lib_Piccolo/Pitch to Elevator/Cm//Alpha Estimation ==
  note: 'Stiffness' here represents the slope of a linearized Cm/Alpha curve. Multiplication against alpha estimate produces an esitmated pitch moment contribution.
  note: This calculation assumes that the Cl/alpha curve crosses (0,0) in clean configuration.
  zAccel_Body : Inport
  Q : Inport  Port=2
  Constant : Constant  Value=PitchStiffness
  Constant1 : Constant  Value=dCl_per_dFlap
  Divide : Product  Inputs=*/
  Divide1 : Product  Inputs=*/
  Gain : Gain  Gain=m/Sw
  LPF CLest : Subsystem
  Lift Slope : Constant  Value=LiftSlope
  Multiply : Product
  Multiply1 : Product
  Sum : Sum  Inputs=-+|
  STIFF : Outport
  tag scope: AoA=global
  wires:
  Divide1/1 -> LPF CLest/1(Input)  "Pic_AoA"
  Sum/1 -> Divide1/1
  Multiply1/1 -> Sum/1
  Constant1/1 -> Multiply1/1
  [flapCmd] -> Multiply1/2
  LPF CLest/1(Output) -> [AoA], Multiply/2  "Pic_AoA_Filtered"
  zAccel_Body/1 -> Gain/1
  Divide/1 -> Sum/2  "Pic_CL"
  Lift Slope/1 -> Divide1/2
  Q/1 -> Divide/2
  Gain/1 -> Divide/1
  Multiply/1 -> STIFF/1  "STIFF"
  Constant/1 -> Multiply/1

== system Lib_Piccolo/Pitch to Elevator/Dimensional Elevator Power ==
  Dynamic Pressure (Avoid Small Value) : Inport
  Average Wing Chord : Constant  Value=c
  Multiply : Product  Inputs=****/
  Unit: Per Deg : Constant  Value=ElevatorPower
  Wing Area : Constant  Value=Sw
  YInertia : Constant  Value=YInertia
  CP : Outport
  wires:
  Unit: Per Deg/1 -> Multiply/4
  Multiply/1 -> CP/1
  YInertia/1 -> Multiply/5
  Average Wing Chord/1 -> Multiply/3
  Wing Area/1 -> Multiply/2
  Dynamic Pressure (Avoid Small Value)/1 -> Multiply/1

== system Lib_Piccolo/Pitch to Elevator/DynamicPLimit ==
  note: Q saturates at ~ 100mps which in IAS is 6125Pa
  apMode : Inport
  DynamicPressure_Pa : Inport  Port=2
  Compare To Constant1 : simulink/Logic and Bit Operations/Compare To Constant  relop=>=  const=5  OutDataTypeStr=uint8
  Compare To Constant2 : simulink/Logic and Bit Operations/Compare To Constant  relop=>=  const=11  OutDataTypeStr=uint8
  Compare To Constant3 : simulink/Logic and Bit Operations/Compare To Constant  relop=>=  const=10  OutDataTypeStr=uint8
  Gain : Gain  Gain=0.5 * 1.225
  Gain1 : Gain  Gain=1.1
  Gain2 : Gain  Gain=0.8
  Gain3 : Gain  Gain=0.5 * 1.225
  Latch : Subsystem
  Qmax : Constant  Value=6125
  Saturation Dynamic : simulink/Discontinuities/Saturation Dynamic  OutMin=[]  OutMax=[]  OutDataTypeStr=Inherit: Same as second input  OutDataType=fixdt(1, 16)  OutScaling=2^-10  DoSatur=off
  Square : Math  Operator=square  SaturateOnIntegerOverflow=on
  Square1 : Math  Operator=square  SaturateOnIntegerOverflow=on
  Switch : Switch  Criteria=u2 > Threshold
  Switch1 : Switch  Criteria=u2 > Threshold
  Out1 : Outport
  tag scope: Qmin=global, Qmin_Bounce=global, Qmin_Flare=global
  wires:
  Square1/1 -> Gain3/1
  [IASmin] -> Square1/1
  Gain/1 -> Gain1/1, Gain2/1
  [IASstall] -> Square/1
  Square/1 -> Gain/1
  Latch/1(Q_Latched) -> Switch1/2
  Switch1/1 -> Saturation Dynamic/3
  Gain2/1 -> Switch1/1, [Qmin_Bounce]  "Qmin_Bounce"
  Switch/1 -> Switch1/3
  Compare To Constant2/1 -> Latch/1(D)
  Compare To Constant1/1 -> Latch/2(Enable/!Rst)
  Qmax/1 -> Saturation Dynamic/1
  Gain1/1 -> Switch/1, [Qmin_Flare]  "Qmin_Flare"
  Gain3/1 -> Switch/3, [Qmin]  "Qmin"
  Compare To Constant3/1 -> Switch/2
  apMode/1 -> Compare To Constant1/1, Compare To Constant2/1, Compare To Constant3/1
  Saturation Dynamic/1 -> Out1/1
  DynamicPressure_Pa/1 -> Saturation Dynamic/2

== system Lib_Piccolo/Pitch to Elevator/Elevator Ramp Logic ==
  Elevator In : Inport
  AP Mode : Inport  Port=2
  Elevator DeRotation Ramp : Subsystem
  Elevator Rotation Ramp : Subsystem
  Elevator Out : Outport
  wires:
  Elevator Rotation Ramp/1(Elevator Out) -> Elevator Out/1
  Elevator DeRotation Ramp/1(Elevator Out) -> Elevator Rotation Ramp/1(Elevator In)
  Elevator In/1 -> Elevator DeRotation Ramp/1(Elevator In)
  AP Mode/1 -> Elevator DeRotation Ramp/2(apMode In), Elevator Rotation Ramp/2(apMode In)

== system Lib_Piccolo/Pitch to Elevator/LPF Elevator ==
  Input : Inport
  Reset : Inport  Port=2
  ResetValue : Inport  Port=3
  Add1 : Sum  Inputs=++|
  Compare To Constant2 : simulink/Logic and Bit Operations/Compare To Constant  relop=>  const=0  OutDataTypeStr=uint8
  Constant11 : Constant  Value=PitchRateLpfCutoff
  Switch : Switch  Criteria=u2 > Threshold
  Switch1 : Switch  Criteria=u2 > Threshold
  Unit Delay1 : UnitDelay  InitialCondition=LPFvRate2PitchInit*pi/180  SampleTime=-1
  a1 : Gain  Gain=1-Fp_Elevator
  b0 : Gain  Gain=Fp_Elevator
  Output : Outport
  wires:
  ResetValue/1 -> Switch/1
  Reset/1 -> Switch/2
  Switch/1 -> Unit Delay1/1
  Input/1 -> b0/1, Switch1/3
  Add1/1 -> Switch1/1, Switch/3
  b0/1 -> Add1/2
  Unit Delay1/1 -> a1/1
  a1/1 -> Add1/1
  Switch1/1 -> Output/1
  Compare To Constant2/1 -> Switch1/2
  Constant11/1 -> Compare To Constant2/1

== system Lib_Piccolo/Pitch to Elevator/Pitch Moment Caused By Damping ==
  note: An estimation of damping moment produced proportionally to body pitch rate.
  PitchRate_Body : Inport
  TAS : Inport  Port=2
  AverageWingChord : Constant  Value=c
  Constant : Constant  Value=PitchDamping
  Gain : Gain  Gain=2
  Multiply : Product  Inputs=***/
  DAMP : Outport
  wires:
  PitchRate_Body/1 -> Multiply/2
  TAS/1 -> Gain/1
  Constant/1 -> Multiply/1
  Multiply/1 -> DAMP/1
  Gain/1 -> Multiply/4
  AverageWingChord/1 -> Multiply/3

== system Lib_Piccolo/Pitch to Elevator/Reference Frame Conversion and Pitch Rate Limit Determination ==
  PitchCmd_Euler : Inport
  Pitch_Euler : Inport  Port=2
  Roll_Euler : Inport  Port=3
  V : Inport  Port=4
  Q : Inport  Port=5
  AeroVsStruct_Limit : Subsystem
  Constant : Constant  Value=PitchRateMax_User
  MATLAB Function : MATLAB Function  TreatAsAtomicUnit=on
  Saturation : Saturate  UpperLimit=100  LowerLimit=5
  Terminator : Terminator
  Terminator1 : Terminator
  PitchCmd_Body : Outport
  "Pitch_Body " : Outport  Port=2
  "Scalar " : Outport  Port=3
  PitchRateCmd_Body : Outport  Port=4
  "PitchRateLimit_Max " : Outport  Port=5
  "PitchRateLimit_Min " : Outport  Port=6
  wires:
  MATLAB Function/8(nPrime_Min) -> Terminator1/1
  MATLAB Function/7(nPrime_Max) -> Terminator/1
  Q/1 -> AeroVsStruct_Limit/1(Q)
  AeroVsStruct_Limit/2("nMin ") -> MATLAB Function/6(nMin)
  AeroVsStruct_Limit/1(nMax) -> MATLAB Function/5(nMax)
  MATLAB Function/4(PitchRateCmd_Body) -> PitchRateCmd_Body/1
  Constant/1 -> MATLAB Function/7(PitchRateMax_User)
  MATLAB Function/6(PitchRateLimit_Min) -> "PitchRateLimit_Min "/1
  MATLAB Function/5(PitchRateLimit_Max) -> "PitchRateLimit_Max "/1
  MATLAB Function/3(Scalar) -> "Scalar "/1
  MATLAB Function/2(Pitch_Body) -> "Pitch_Body "/1
  MATLAB Function/1(PitchCmd_Body) -> PitchCmd_Body/1
  Roll_Euler/1 -> MATLAB Function/3(Roll_Euler)
  Pitch_Euler/1 -> MATLAB Function/2(Pitch_Euler)
  PitchCmd_Euler/1 -> MATLAB Function/1(PitchCmd_Euler)
  V/1 -> Saturation/1
  Saturation/1 -> MATLAB Function/4(V)

== system Lib_Piccolo/Pitch to Elevator/TASLimit ==
  note: TAS saturates at ~ 100mps which in IAS is 6125Pa
  apMode : Inport
  <V_mps> : Inport  Port=2
  Compare To Constant1 : simulink/Logic and Bit Operations/Compare To Constant  relop=>=  const=5  OutDataTypeStr=uint8
  Compare To Constant2 : simulink/Logic and Bit Operations/Compare To Constant  relop=>=  const=11  OutDataTypeStr=uint8
  Compare To Constant4 : simulink/Logic and Bit Operations/Compare To Constant  relop=>=  const=10  OutDataTypeStr=uint8
  Gain : Gain  Gain=0.8
  Latch : Subsystem
  Saturation Dynamic1 : simulink/Discontinuities/Saturation Dynamic  OutMin=[]  OutMax=[]  OutDataTypeStr=Inherit: Same as second input  OutDataType=fixdt(1, 16)  OutScaling=2^-10  DoSatur=off
  Switch1 : Switch  Criteria=u2 > Threshold
  Switch2 : Switch  Criteria=u2 > Threshold
  TASmax : Constant  Value=100
  Out1 : Outport
  wires:
  TASmax/1 -> Saturation Dynamic1/1
  Gain/1 -> Switch2/1  "IASbounce"
  Compare To Constant1/1 -> Latch/2(Enable/!Rst)
  Switch1/1 -> Switch2/3
  apMode/1 -> Compare To Constant4/1, Compare To Constant2/1, Compare To Constant1/1
  Compare To Constant2/1 -> Latch/1(D)
  Latch/1(Q_Latched) -> Switch2/2
  <V_mps>/1 -> Saturation Dynamic1/2
  [IASmin] -> Switch1/3
  Saturation Dynamic1/1 -> Out1/1
  [IASstall] -> Switch1/1, Gain/1
  Compare To Constant4/1 -> Switch1/2
  Switch2/1 -> Saturation Dynamic1/3

== system Lib_Piccolo/Pitch to Elevator/Triggered Subsystem ==
  In1 : Inport
  Trigger : TriggerPort  TriggerType=falling  VariantControl=Variant
  Out1 : Outport
  wires:
  In1/1 -> Out1/1

== system Lib_Piccolo/Pitch to Elevator/resetCondition ==
  Compare To Constant1 : simulink/Logic and Bit Operations/Compare To Constant  relop=<=  const=2  OutDataTypeStr=uint8
  Compare To Constant3 : simulink/Logic and Bit Operations/Compare To Constant  relop===  const=11  OutDataTypeStr=uint8
  NOT : Logic  Operator=NOT  IconShape=distinctive  AllPortsSameDT=off  OutDataTypeStr=boolean
  OR : Logic  Operator=OR  Inputs=3  IconShape=distinctive  AllPortsSameDT=off  OutDataTypeStr=boolean
  reset : Outport
  wires:
  NOT/1 -> OR/3
  [ApGlobal] -> NOT/1
  Compare To Constant1/1 -> OR/2
  OR/1 -> reset/1  "Sim.KI_Pitch_Reset"
  Compare To Constant3/1 -> OR/1
  [Pic_AP_Mode] -> Compare To Constant3/1, Compare To Constant1/1

== system Lib_Piccolo/Pitch to Elevator/resetVal ==
  note: This init value is intended to aid trimming at start of in-flight simulation and should not be used for reset during liftoffs/bouncing. Will use 0 as alternative reset value as was done previously
  Constant1 : Constant  Value=Pitch2ElevatorIntegratorInit
  Constant2 : Constant  Value=0
  Constant3 : Constant  Value=0
  Switch : Switch  Threshold=9
  Switch1 : Switch  Threshold=3
  resetVal : Outport
  wires:
  Constant3/1 -> Switch1/3
  Switch1/1 -> Switch/3
  Constant1/1 -> Switch1/1
  Switch/1 -> resetVal/1
  [Pic_AP_Mode] -> Switch/2, Switch1/2
  Constant2/1 -> Switch/1

== system Lib_Piccolo/REF INS Replay/Slope Vz Calculation ==
  VGround : Inport
  apMode : Inport  Port=2
  Compare To Constant : simulink/Logic and Bit Operations/Compare To Constant  relop=>=  const=5  OutDataTypeStr=boolean
  Compare To Constant1 : simulink/Logic and Bit Operations/Compare To Constant  relop=>=  const=9  OutDataTypeStr=boolean
  Constant13 : Constant  Value=FinalDescentSlope_Deg*pi/180
  Constant14 : Constant  Value=ShortDescentSlope_Deg*pi/180
  CruiseSlope_Deg : Constant  Value=0
  Gain : Gain  Gain=-1
  Multiply10 : Product
  Sin3 : Trigonometry
  Switch3 : Switch  Criteria=u2 > Threshold
  Switch4 : Switch  Criteria=u2 > Threshold
  Vz_Cmd : Outport
  wires:
  Compare To Constant/1 -> Switch4/2
  Compare To Constant1/1 -> Switch3/2
  Switch4/1 -> Sin3/1
  Gain/1 -> Multiply10/1
  Constant13/1 -> Switch3/3
  VGround/1 -> Gain/1
  CruiseSlope_Deg/1 -> Switch4/3
  Multiply10/1 -> Vz_Cmd/1
  Constant14/1 -> Switch3/1
  Sin3/1 -> Multiply10/2
  Switch3/1 -> Switch4/1
  apMode/1 -> Compare To Constant1/1, Compare To Constant/1

== system Lib_Piccolo/Steering Controller Landing/Nosegear rudder mixer  ==
  "Desired nosegear " : Inport
  NoseGear2Rudder : Gain  Gain=AutoNosegear2Rudder
  Saturation : Saturate  UpperLimit=ldg_NosegearMax  LowerLimit=-ldg_NosegearMax
  Saturation1 : Saturate  UpperLimit=RudderMax  LowerLimit=-RudderMax
  rad2deg : Gain  Gain=180/pi
  Nosegear command : Outport
  Rudder command : Outport  Port=2
  wires:
  rad2deg/1 -> Saturation/1, NoseGear2Rudder/1
  "Desired nosegear "/1 -> rad2deg/1
  NoseGear2Rudder/1 -> Saturation1/1
  Saturation/1 -> Nosegear command/1
  Saturation1/1 -> Rudder command/1

== system Lib_Piccolo/Steering Controller Landing/Nosegear scaling based on ground speed ==
  Ground Speed : Inport
  "Vy to nosegear scaling " : Inport  Port=2
  Divide : Product  Inputs=*/
  SteeringArm : Constant  Value=SteeringArm
  Vy Scalar1 : Math  Operator=pow  SaturateOnIntegerOverflow=on
  nosegear scalar : Outport
  wires:
  "Vy to nosegear scaling "/1 -> Vy Scalar1/2
  Divide/1 -> nosegear scalar/1
  SteeringArm/1 -> Divide/1
  Vy Scalar1/1 -> Divide/2
  Ground Speed/1 -> Vy Scalar1/1

== system Lib_Piccolo/Steering Controller Landing/Vy scaling based on ground speed ==
  Ground Speed : Inport
  Y to Vy scaling power : Inport  Port=2
  Power Function : Math  Operator=pow  SaturateOnIntegerOverflow=on
  Vy Scalar : Outport
  wires:
  Y to Vy scaling power/1 -> Power Function/2
  Ground Speed/1 -> Power Function/1
  Power Function/1 -> Vy Scalar/1

== system Lib_Piccolo/Steering Controller Transition/Nosegear rudder mixer  ==
  "Desired nosegear " : Inport
  NoseGear2Rudder : Gain  Gain=AutoNosegear2Rudder
  Saturation : Saturate  UpperLimit=NosegearMax  LowerLimit=-NosegearMax
  Saturation1 : Saturate  UpperLimit=RudderMax  LowerLimit=-RudderMax
  rad2deg : Gain  Gain=180/pi
  Nosegear command : Outport
  Rudder command : Outport  Port=2
  wires:
  rad2deg/1 -> Saturation/1, NoseGear2Rudder/1
  "Desired nosegear "/1 -> rad2deg/1
  NoseGear2Rudder/1 -> Saturation1/1
  Saturation/1 -> Nosegear command/1
  Saturation1/1 -> Rudder command/1

== system Lib_Piccolo/Steering Controller Transition/Nosegear scaling based on ground speed ==
  Ground Speed : Inport
  "Vy to nosegear scaling " : Inport  Port=2
  Divide : Product  Inputs=*/
  SteeringArm : Constant  Value=SteeringArm
  Vy Scalar1 : Math  Operator=pow  SaturateOnIntegerOverflow=on
  nosegear scalar : Outport
  wires:
  "Vy to nosegear scaling "/1 -> Vy Scalar1/2
  Divide/1 -> nosegear scalar/1
  SteeringArm/1 -> Divide/1
  Vy Scalar1/1 -> Divide/2
  Ground Speed/1 -> Vy Scalar1/1

== system Lib_Piccolo/Steering Controller Transition/Vy scaling based on ground speed ==
  Ground Speed : Inport
  Y to Vy scaling power : Inport  Port=2
  Power Function : Math  Operator=pow  SaturateOnIntegerOverflow=on
  Vy Scalar : Outport
  wires:
  Y to Vy scaling power/1 -> Power Function/2
  Ground Speed/1 -> Power Function/1
  Power Function/1 -> Vy Scalar/1
